simulink model "EndEffectorVSCube_v2"  (Simulink 7.4)
settings: Solver=FixedStepDiscrete  StartTime=0.0  StopTime=80  FixedStep=dt  RelTol=1e-3
InitFcn:
  | start_EEVSCube2
undefined symbols (not defined in the file or in its folder): DiscIntNeverNeededParam, dt, mesh_A, mesh_B
libraries: simulink x2, dspsigops x1
settings Model: Creator=SIMONE  LastModifiedBy=Administrator
settings SolverCC: PositivePriorityOrder=on
settings DataIOCC: LimitDataPoints=off  SaveOutput=off  SignalLogging=off
settings RTWCC: GenerateMakefile=off

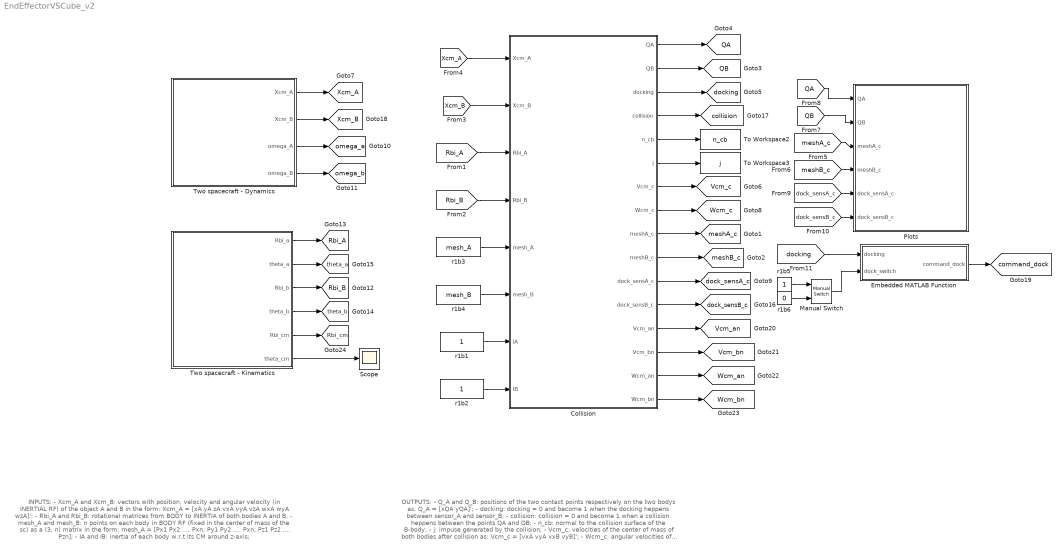
== system EndEffectorVSCube_v2 ==
  note: INPUTS:
      | - Xcm_A and Xcm_B: vectors with position, velocity and angular velocity (in INERTIAL RF)
      |                                        of the object A and B in the form:
      |                                        Xcm_A = [xA yA zA vxA vyA vzA wxA wyA wzA]';
      | - Rbi_A and Rbi_B: rotational matrices from BODY to INERTIA of both bodies A and B;
      | - mesh_A and mesh_B: n points on each body in BODY RF (fixed in the center of mass
      |                                          of the sc) as a (3, n) matrix in the form:
      |                                          mesh_A = [Px1 Px2 .... Pxn;
      |                                                             Py1 Py2 .... Pxn;
      |                                                             Pz1 Pz2 .... Pzn];
      | - IA and IB: inertia of each body w.r.t its CM around z-axis;
  note: OUTPUTS:
      | - Q_A and Q_B: positions of the two contact points respectively on the two bodys as,
      |                              Q_A = [xQA yQA]';
      | - docking: docking = 0 and become 1 when the docking heppens between sensor_A and sensor_B;
      | - collision: collision = 0 and become 1 when a collision heppens between the points QA and QB;
      | - n_cb: normal to the collision surface of the B-body;
      | - j: impuse generated by the collision;
      | - Vcm_c: velocities of the center of mass of both bodies after collision as:
      |                  Vcm_c = [vxA vyA vxB vyB]';
      | - Wcm_c: angular velocities of the center of mass of both bodies after collision as:
      |                    Wcm_c = [wxA wyA wxB wyB]'.
      | - meshA_c and meshB_c: n points on each body in INERTIAL RF propagated during the simulation,
      |                                                     as a (1, 3*n) vector in the form:
      |                                                      pointsA_c = [Px1 Py1 Px2 Py2 .... Pxn Pyn];
      | - dock_sensA_c and dock_sensB_c: position of the docking sensors on A and B in INERTIAL RF while simulation is running;
  Collision : Subsystem  mask{mA=1e6, mB=1, sigma=0.01, sigma_dock=0.1, dotsigma_dock=1, dock_sensA=[0.5 0 0]', dock_sensB=[-0.5 0 0]', epsilon=1}
      mask prompts: mA "Mass of body A [Kg]"; mB "Mass of body B [Kg]"; sigma "Minimum distance for contact [m]"; sigma_dock "Minimum distance for docking (must be greater than contact distance) [m]"; dotsigma_dock "Maximum relative velocity for docking [m/s]"; dock_sensA "Docking sensor position (Body RF) on body A (as [x y z]') [m]"; dock_sensB "Docking sensor position (Body RF) on body B (as [x y z]') [m]"; epsilon "Coefficent of restitution"
      mask help: This block implements collision detection and responce for two rigid bodies of general shapes.
      mask init:
      | ma_mb = [mA; 
      |          mB];
      mask Display:
      | image(imread('collision.jpeg'))
      | color('red');
      | disp('Collision \n Detection and Responce \n v.1.0.9')
      | port_label('input',1,'Xcm_A')
      | port_label('input',2,'Xcm_B')
      | port_label('input',3,'Rbi_A')
      | port_label('input',4,'Rbi_B')
      | port_label('input',5,'mesh_A')
      | port_label('input',6,'mesh_B')
      | port_label('input',7,'IA')
      | port_label('input',8,'IB')
      | 
      | port_label('output',1,'QA')
      | port_label('output',2,'QB')
      | port_label('output',3,'docking')
      | port_label('output',4,'collision')
      | port_label('output',5,'n_cb')
      | port_label('output',6,'j')
      | port_label('output',7,'Vcm_c')
      | port_label('output',8,'Wcm_c')
      | port_label('output',9,'meshA_c')
      | port_label('output',10,'meshB_c')
      | port_label('output',11,'dock_sensA_c')
      | port_label('output',12,'dock_sensB_c')
      | port_label('output',13,'Vcm_an')
      | port_label('output',14,'Vcm_bn')
      | port_label('output',15,'Wcm_an')
      | port_label('output',16,'Wcm_bn')
  Embedded MATLAB Function : Stateflow chart  TreatAsAtomicUnit=on
  Manual Switch : simulink/Signal Routing/Manual Switch  SystemSampleTime=-1  sw=1  action=0  varsize=off
  Plots : Subsystem
  Scope : Scope
      settings: TimeRange=3  YMin=-1  YMax=1.5  SaveName=ScopeData3
  To Workspace2 : ToWorkspace  VariableName=n_cb  SampleTime=-1  SaveFormat=Array
  To Workspace3 : ToWorkspace  VariableName=j  SampleTime=-1  SaveFormat=Array
  Two spacecraft - Dynamics : Subsystem
  Two spacecraft - Kinematics : Subsystem
  r1b1 : Constant
  r1b2 : Constant
  r1b3 : Constant  Value=mesh_A
  r1b4 : Constant  Value=mesh_B
  r1b5 : Constant
  r1b6 : Constant  Value=0
  tag scope: QA=global, QB=global, Rbi_A=global, Rbi_B=global, Rbi_cm=global, Vcm_an=global, Vcm_bn=global, Vcm_c=global, Wcm_an=global, Wcm_bn=global, Wcm_c=global, Xcm_A=global, Xcm_B=global, collision=global, command_dock=global, dock_sensA_c=global, dock_sensB_c=global, docking=global, meshA_c=global, meshB_c=global, omega_a=global, omega_b=global, theta_a=global, theta_b=global
  wires:
  Collision/1(QA) -> [QA]
  Collision/2(QB) -> [QB]
  Collision/3(docking) -> [docking]
  Two spacecraft - Dynamics/3(omega_A) -> [omega_a]
  Two spacecraft - Dynamics/4(omega_B) -> [omega_b]
  Two spacecraft - Dynamics/1(Xcm_A) -> [Xcm_A]
  Two spacecraft - Kinematics/3(Rbi_b) -> [Rbi_B]
  Two spacecraft - Kinematics/1(Rbi_a) -> [Rbi_A]
  Two spacecraft - Kinematics/2(theta_a) -> [theta_a]
  Two spacecraft - Kinematics/4(theta_b) -> [theta_b]
  Collision/6(j) -> To Workspace3/1
  Collision/4(collision) -> [collision]
  Two spacecraft - Dynamics/2(Xcm_B) -> [Xcm_B]
  [Xcm_A] -> Collision/1(Xcm_A)
  [Xcm_B] -> Collision/2(Xcm_B)
  [Rbi_A] -> Collision/3(Rbi_A)
  [Rbi_B] -> Collision/4(Rbi_B)
  r1b3/1 -> Collision/5(mesh_A)
  r1b4/1 -> Collision/6(mesh_B)
  Collision/5(n_cb) -> To Workspace2/1
  Collision/7(Vcm_c) -> [Vcm_c]
  Collision/8(Wcm_c) -> [Wcm_c]
  Collision/9(meshA_c) -> [meshA_c]
  Collision/10(meshB_c) -> [meshB_c]
  [QA] -> Plots/1(QA)
  [QB] -> Plots/2(QB)
  [meshA_c] -> Plots/3(meshA_c)
  [meshB_c] -> Plots/4(meshB_c)
  Collision/11(dock_sensA_c) -> [dock_sensA_c]
  Collision/12(dock_sensB_c) -> [dock_sensB_c]
  [dock_sensA_c] -> Plots/5(dock_sensA_c)
  [dock_sensB_c] -> Plots/6(dock_sensB_c)
  r1b1/1 -> Collision/7(IA)
  r1b2/1 -> Collision/8(IB)
  [docking] -> Embedded MATLAB Function/1(docking)
  Embedded MATLAB Function/1(command_dock) -> [command_dock]
  Manual Switch/1 -> Embedded MATLAB Function/2(dock_switch)
  r1b5/1 -> Manual Switch/1
  r1b6/1 -> Manual Switch/2
  Collision/13(Vcm_an) -> [Vcm_an]
  Collision/14(Vcm_bn) -> [Vcm_bn]
  Collision/15(Wcm_an) -> [Wcm_an]
  Collision/16(Wcm_bn) -> [Wcm_bn]
  Two spacecraft - Kinematics/5(Rbi_cm) -> [Rbi_cm]
  Two spacecraft - Kinematics/6(theta_cm) -> Scope/1

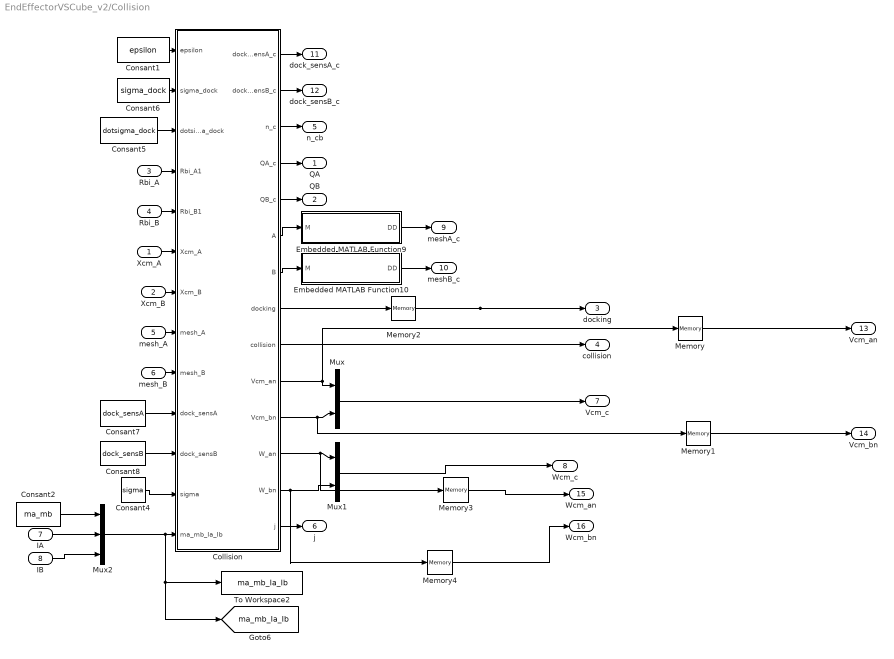
== system EndEffectorVSCube_v2/Collision ==
  Xcm_A : Inport
  Xcm_B : Inport  Port=2
  Rbi_A : Inport  Port=3
  Rbi_B : Inport  Port=4
  mesh_A : Inport  Port=5
  mesh_B : Inport  Port=6
  IA : Inport  Port=7
  IB : Inport  Port=8
  Collision : Stateflow chart  TreatAsAtomicUnit=on
  Consant1 : Constant  Value=epsilon
  Consant2 : Constant  Value=ma_mb
  Consant4 : Constant  Value=sigma
  Consant5 : Constant  Value=dotsigma_dock
  Consant6 : Constant  Value=sigma_dock
  Consant7 : Constant  Value=dock_sensA
  Consant8 : Constant  Value=dock_sensB
  Embedded MATLAB Function10 : Stateflow chart  TreatAsAtomicUnit=on
  Embedded MATLAB Function9 : Stateflow chart  TreatAsAtomicUnit=on
  Memory{,1,3..4} (4 alike) : Memory  X0=zeros(3,1)
  Memory2 : Memory
  Mux : Mux  Inputs=2
  Mux1 : Mux  Inputs=2
  Mux2 : Mux  Inputs=3
  To Workspace2 : ToWorkspace  VariableName=ma_mb_Ia_Ib  SampleTime=-1  SaveFormat=Array
  QA : Outport
  QB : Outport  Port=2
  docking : Outport  Port=3
  collision : Outport  Port=4
  n_cb : Outport  Port=5
  j : Outport  Port=6
  Vcm_c : Outport  Port=7
  Wcm_c : Outport  Port=8
  meshA_c : Outport  Port=9
  meshB_c : Outport  Port=10
  dock_sensA_c : Outport  Port=11
  dock_sensB_c : Outport  Port=12
  Vcm_an : Outport  Port=13
  Vcm_bn : Outport  Port=14
  Wcm_an : Outport  Port=15
  Wcm_bn : Outport  Port=16
  tag scope: ma_mb_Ia_Ib=global
  wires:
  Embedded MATLAB Function9/1(DD) -> meshA_c/1
  Embedded MATLAB Function10/1(DD) -> meshB_c/1
  Collision/6(A) -> Embedded MATLAB Function9/1(M)
  Collision/7(B) -> Embedded MATLAB Function10/1(M)
  Rbi_B/1 -> Collision/5(Rbi_B1)
  Xcm_A/1 -> Collision/6(Xcm_A)
  mesh_A/1 -> Collision/8(mesh_A)
  mesh_B/1 -> Collision/9(mesh_B)
  Collision/3(n_c) -> n_cb/1
  Collision/8(docking) -> Memory2/1
  Collision/10(Vcm_an) -> Mux/1, Memory/1
  Collision/13(W_bn) -> Mux1/2, Memory4/1
  Collision/14(j) -> j/1
  Collision/9(collision) -> collision/1
  Mux/1 -> Vcm_c/1
  Mux1/1 -> Wcm_c/1
  Collision/4(QA_c) -> QA/1
  Collision/5(QB_c) -> QB/1
  Collision/11(Vcm_bn) -> Memory1/1, Mux/2
  Collision/12(W_an) -> Memory3/1, Mux1/1
  Xcm_B/1 -> Collision/7(Xcm_B)
  Collision/2(dock_sensB_c) -> dock_sensB_c/1
  Collision/1(dock_sensA_c) -> dock_sensA_c/1
  Consant4/1 -> Collision/12(sigma)
  Consant5/1 -> Collision/3(dotsigma_dock)
  Rbi_A/1 -> Collision/4(Rbi_A1)
  Consant6/1 -> Collision/2(sigma_dock)
  Consant7/1 -> Collision/10(dock_sensA)
  Consant8/1 -> Collision/11(dock_sensB)
  Consant1/1 -> Collision/1(epsilon)
  Mux2/1 -> Collision/13(ma_mb_Ia_Ib), To Workspace2/1, [ma_mb_Ia_Ib]
  Consant2/1 -> Mux2/1
  IA/1 -> Mux2/2
  IB/1 -> Mux2/3
  Memory/1 -> Vcm_an/1
  Memory1/1 -> Vcm_bn/1
  Memory3/1 -> Wcm_an/1
  Memory4/1 -> Wcm_bn/1
  Memory2/1 -> docking/1

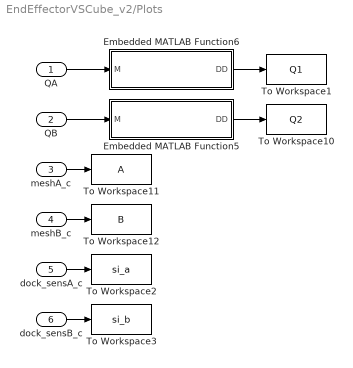
== system EndEffectorVSCube_v2/Plots ==
  QA : Inport
  QB : Inport  Port=2
  meshA_c : Inport  Port=3
  meshB_c : Inport  Port=4
  dock_sensA_c : Inport  Port=5
  dock_sensB_c : Inport  Port=6
  Embedded MATLAB Function5 : Stateflow chart  TreatAsAtomicUnit=on
  Embedded MATLAB Function6 : Stateflow chart  TreatAsAtomicUnit=on
  To Workspace1 : ToWorkspace  VariableName=Q1  SampleTime=-1  SaveFormat=Array
  To Workspace10 : ToWorkspace  VariableName=Q2  SampleTime=-1  SaveFormat=Array
  To Workspace11 : ToWorkspace  VariableName=A  SampleTime=-1  SaveFormat=Array
  To Workspace12 : ToWorkspace  VariableName=B  SampleTime=-1  SaveFormat=Array
  To Workspace2 : ToWorkspace  VariableName=si_a  SampleTime=-1  SaveFormat=Array
  To Workspace3 : ToWorkspace  VariableName=si_b  SampleTime=-1  SaveFormat=Array
  wires:
  Embedded MATLAB Function6/1(DD) -> To Workspace1/1
  Embedded MATLAB Function5/1(DD) -> To Workspace10/1
  QA/1 -> Embedded MATLAB Function6/1(M)
  QB/1 -> Embedded MATLAB Function5/1(M)
  meshB_c/1 -> To Workspace12/1
  meshA_c/1 -> To Workspace11/1
  dock_sensA_c/1 -> To Workspace2/1
  dock_sensB_c/1 -> To Workspace3/1

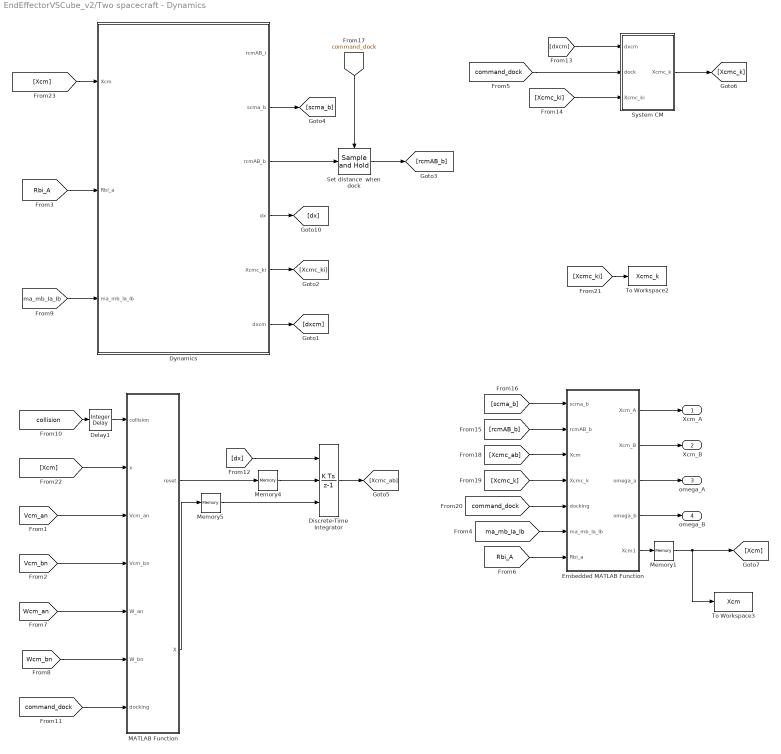
== system EndEffectorVSCube_v2/Two spacecraft - Dynamics ==
  Delay1 : simulink/Discrete/Integer Delay  vinit=0  samptime=-1  NumDelays=1
  Discrete-Time Integrator : DiscreteIntegrator  ExternalReset=rising  InitialConditionSource=external  SampleTime=dt  ICPrevOutput=DiscIntNeverNeededParam  ICPrevScaledInput=DiscIntNeverNeededParam
  Dynamics : Stateflow chart  TreatAsAtomicUnit=on
  Embedded MATLAB Function : Stateflow chart  TreatAsAtomicUnit=on
  MATLAB Function : Stateflow chart  TreatAsAtomicUnit=on
  Memory1 : Memory  X0=zeros(10,1)
  Memory4 : Memory
  Memory5 : Memory  X0=[-1, 0, 0, 0, 0, 2.5*2, 0, -0.2, 0, -0.2]'
  Set distance  when dock : dspsigops/Sample and Hold  SystemSampleTime=-1  trig=Rising edge  initCond=0  latchinput=off
  System CM : Subsystem
  To Workspace2 : ToWorkspace  VariableName=Xcmc_k  SampleTime=-1  SaveFormat=Array
  To Workspace3 : ToWorkspace  VariableName=Xcm  SampleTime=-1  SaveFormat=Array
  Xcm_A : Outport  PortDimensions=[9,1]
  Xcm_B : Outport  Port=2  PortDimensions=[9,1]
  omega_A : Outport  Port=3
  omega_B : Outport  Port=4
  wires:
  [Rbi_A] -> Dynamics/2(Rbi_a)
  Embedded MATLAB Function/1(Xcm_A) -> Xcm_A/1
  Embedded MATLAB Function/2(Xcm_B) -> Xcm_B/1
  MATLAB Function/2(X) -> Memory5/1
  Memory5/1 -> Discrete-Time Integrator/3
  MATLAB Function/1(reset) -> Memory4/1
  Embedded MATLAB Function/3(omega_a) -> omega_A/1
  Embedded MATLAB Function/4(omega_b) -> omega_B/1
  [Vcm_an] -> MATLAB Function/3(Vcm_an)
  [Vcm_bn] -> MATLAB Function/4(Vcm_bn)
  [collision] -> Delay1/1
  Memory4/1 -> Discrete-Time Integrator/2
  [Wcm_an] -> MATLAB Function/5(W_an)
  [Wcm_bn] -> MATLAB Function/6(W_bn)
  [ma_mb_Ia_Ib] -> Dynamics/3(ma_mb_Ia_Ib)
  [ma_mb_Ia_Ib] -> Embedded MATLAB Function/6(ma_mb_Ia_Ib)
  Delay1/1 -> MATLAB Function/1(collision)
  [command_dock] -> System CM/2(dock)
  [Rbi_A] -> Embedded MATLAB Function/7(Rbi_a)
  Embedded MATLAB Function/5(Xcm1) -> Memory1/1
  Dynamics/4(dx) -> [dx]
  [dx] -> Discrete-Time Integrator/1
  Dynamics/6(dxcm) -> [dxcm]
  [dxcm] -> System CM/1(dxcm)
  Dynamics/5(Xcmc_ki) -> [Xcmc_ki]
  [Xcmc_ki] -> System CM/3(Xcmc_ki)
  [rcmAB_b] -> Embedded MATLAB Function/2(rcmAB_b)
  [scma_b] -> Embedded MATLAB Function/1(scma_b)
  Dynamics/2(scma_b) -> [scma_b]
  [command_dock] -> Set distance  when dock/Trigger
  Set distance  when dock/1 -> [rcmAB_b]
  Dynamics/3(rcmAB_b) -> Set distance  when dock/1
  Discrete-Time Integrator/1 -> [Xcmc_ab]
  [Xcmc_ab] -> Embedded MATLAB Function/3(Xcm)
  System CM/1(Xcmc_k) -> [Xcmc_k]
  [Xcmc_k] -> Embedded MATLAB Function/4(Xcmc_k)
  [command_dock] -> Embedded MATLAB Function/5(docking)
  [Xcmc_ki] -> To Workspace2/1
  [Xcm] -> MATLAB Function/2(x)
  [Xcm] -> Dynamics/1(Xcm)
  Memory1/1 -> [Xcm], To Workspace3/1
  [command_dock] -> MATLAB Function/7(docking)

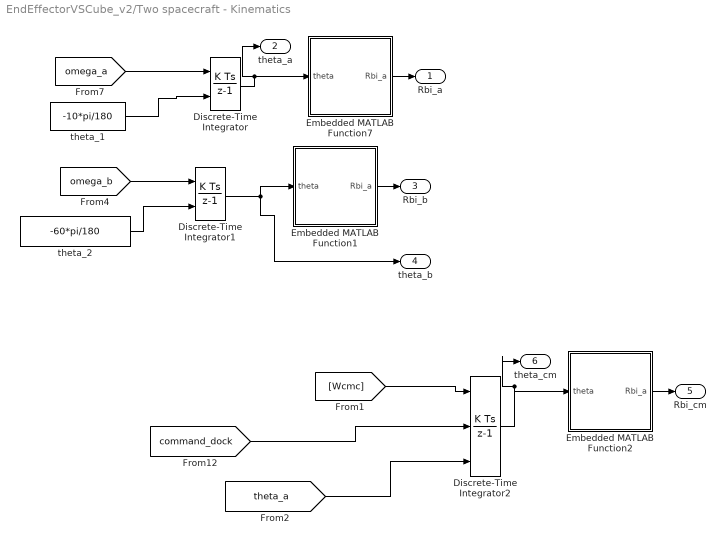
== system EndEffectorVSCube_v2/Two spacecraft - Kinematics ==
  Discrete-Time Integrator : DiscreteIntegrator  InitialConditionSource=external  SampleTime=dt  ICPrevOutput=DiscIntNeverNeededParam  ICPrevScaledInput=DiscIntNeverNeededParam
  Discrete-Time Integrator1 : DiscreteIntegrator  InitialConditionSource=external  SampleTime=dt  ICPrevOutput=DiscIntNeverNeededParam  ICPrevScaledInput=DiscIntNeverNeededParam
  Discrete-Time Integrator2 : DiscreteIntegrator  ExternalReset=rising  InitialConditionSource=external  SampleTime=dt  ICPrevOutput=DiscIntNeverNeededParam  ICPrevScaledInput=DiscIntNeverNeededParam
  Embedded MATLAB Function1 : Stateflow chart  TreatAsAtomicUnit=on
  Embedded MATLAB Function2 : Stateflow chart  TreatAsAtomicUnit=on
  Embedded MATLAB Function7 : Stateflow chart  TreatAsAtomicUnit=on
  theta_1 : Constant  Value=-10*pi/180
  theta_2 : Constant  Value=-60*pi/180
  Rbi_a : Outport  PortDimensions=[2,2]
  theta_a : Outport  Port=2
  Rbi_b : Outport  Port=3  PortDimensions=[2,2]
  theta_b : Outport  Port=4
  Rbi_cm : Outport  Port=5  PortDimensions=[2,2]
  theta_cm : Outport  Port=6
  wires:
  [omega_a] -> Discrete-Time Integrator/1
  theta_1/1 -> Discrete-Time Integrator/2
  Embedded MATLAB Function7/1(Rbi_a) -> Rbi_a/1
  Embedded MATLAB Function1/1(Rbi_a) -> Rbi_b/1
  Discrete-Time Integrator/1 -> theta_a/1, Embedded MATLAB Function7/1(theta)
  Discrete-Time Integrator1/1 -> Embedded MATLAB Function1/1(theta), theta_b/1
  [omega_b] -> Discrete-Time Integrator1/1
  theta_2/1 -> Discrete-Time Integrator1/2
  [Wcmc] -> Discrete-Time Integrator2/1
  Embedded MATLAB Function2/1(Rbi_a) -> Rbi_cm/1
  Discrete-Time Integrator2/1 -> Embedded MATLAB Function2/1(theta), theta_cm/1
  [command_dock] -> Discrete-Time Integrator2/2
  [theta_a] -> Discrete-Time Integrator2/3

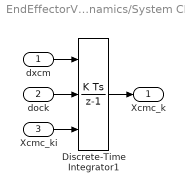
== system EndEffectorVSCube_v2/Two spacecraft - Dynamics/System CM ==
  dxcm : Inport
  dock : Inport  Port=2
  Xcmc_ki : Inport  Port=3
  Discrete-Time Integrator1 : DiscreteIntegrator  ExternalReset=rising  InitialConditionSource=external  SampleTime=dt  ICPrevOutput=DiscIntNeverNeededParam  ICPrevScaledInput=DiscIntNeverNeededParam
  Xcmc_k : Outport
  wires:
  dxcm/1 -> Discrete-Time Integrator1/1
  dock/1 -> Discrete-Time Integrator1/2
  Discrete-Time Integrator1/1 -> Xcmc_k/1
  Xcmc_ki/1 -> Discrete-Time Integrator1/3

== matlab function Two spacecraft - Dynamics/Embedded MATLAB Function ==
  data: scma_b input double; Xcm_A output double; Xcm_B output double; omega_a output double; omega_b output double; Xcm1 output double; rcmAB_b input double; Xcm input double; Xcmc_k input double; docking input double; ma_mb_Ia_Ib input double; Rbi_a input double
function [Xcm_A, Xcm_B,omega_a,omega_b,Xcm1]  = fcn(scma_b,rcmAB_b,Xcm,Xcmc_k, docking, ma_mb_Ia_Ib,Rbi_a)
ma=ma_mb_Ia_Ib(1);
mb=ma_mb_Ia_Ib(2);
Ia=ma_mb_Ia_Ib(3);
Ib=ma_mb_Ia_Ib(4);
% Xcm_B=zeros(9,1);
% Xcm_A=zeros(9,1);

% omega_a=0;
% omega_b=0;
%rcmAB_b=zeros(3,1);

omega_a=Xcm(5);
omega_b=Xcm(10);

xyA = Xcm(1:2);
dxyA = Xcm(3:4);
wA = Xcm(5);

xyB= Xcm(6:7);
dxyB = Xcm(8:9);
wB = Xcm(10);


Xcm_A = [xyA;
         0;
         dxyA;
         0;
         0;
         0;
         wA];
     
Xcm_B = [xyB;
          0;
          dxyB;
          0;
          0;
          0;
          wB];
      
      Xcm1=Xcm;
      
if(docking == 1)
    
    rcm_tot=Xcmc_k(1:2,1);
    vcm_tot=[Xcmc_k(3:4,1); 0];
    %scma_b=[0.5 0 0]';
    wcm_tot=[0 0 Xcmc_k(5)]';
   
    Rbi_a_3=[Rbi_a zeros(2,1)
           0 0 1];
    scma_i=Rbi_a_3*scma_b;
    %body A   
    
    xya=rcm_tot+Rbi_a*scma_b(1:2,1);
    dxya=vcm_tot+cross(wcm_tot,scma_i);
    wa=wcm_tot(3);
    
    %body B
    rcmAB_i=Rbi_a_3*rcmAB_b;
    xyb=xya+rcmAB_i(1:2,1);
    dxyb=dxya+cross(wcm_tot,rcmAB_i);
    wb=wa;
    
    
    
    Xcm_A = [xya;
         0;
         dxya;
         0;
         0;
         wa];
    
       Xcm_B = [xyb;
         0;
         dxyb;
         0;
         0;
         wb];
     
     Xcm1=[xya;
         dxya(1:2);
         wa;
         xyb;
         dxyb(1:2);
         wb];
 omega_a=wa;
omega_b=wb;
    

   
end

== matlab function Collision/Collision ==
  data: epsilon input double; dock_sensA_c output double; dock_sensB_c output double; n_c output double; QA_c output double; QB_c output double; sigma_dock input double; dotsigma_dock input double; Rbi_A1 input double; Rbi_B1 input double; A output double; B output double; Xcm_A input double; Xcm_B input double; mesh_A input double; mesh_B input double; dock_sensA input double; dock_sensB input double; sigma input double; docking output double; ma_mb_Ia_Ib input double; collision output double; Vcm_an output double; Vcm_bn output double; W_an output double; W_bn output double; j output double
function [dock_sensA_c,dock_sensB_c,n_c,QA_c,QB_c,A,B,docking,collision,Vcm_an,Vcm_bn,W_an,W_bn,j] = fcn(epsilon,sigma_dock,dotsigma_dock,Rbi_A1,Rbi_B1,Xcm_A,Xcm_B,mesh_A,mesh_B,dock_sensA,dock_sensB,sigma,ma_mb_Ia_Ib)

[dock_sensA_c,dock_sensB_c,n_c,QA_c,QB_c,A,B,docking,collision,Vcm_an,Vcm_bn,W_an,W_bn,j] = collision_function(epsilon,sigma_dock,dotsigma_dock,Rbi_A1,Rbi_B1,Xcm_A,Xcm_B,mesh_A,mesh_B,dock_sensA,dock_sensB,sigma,ma_mb_Ia_Ib);

== matlab function Two spacecraft - Kinematics/Embedded MATLAB Function1 ==
  data: theta input double; Rbi_a output double
function Rbi_a   = fcn(theta)
%%Defining point 
Rib=[cos(theta) sin(theta)
    -sin(theta) cos(theta)];
Rbi_a=Rib';

== matlab function Two spacecraft - Dynamics/Dynamics ==
  data: rcmAB_i output double; scma_b output double; rcmAB_b output double; Xcm input double; Rbi_a input double; dx output double; Xcmc_ki output double; ma_mb_Ia_Ib input double; dxcm output double
function [rcmAB_i,scma_b,rcmAB_b, dx,Xcmc_ki,dxcm]  = fcn(Xcm, Rbi_a, ma_mb_Ia_Ib)

ma=ma_mb_Ia_Ib(1);
mb=ma_mb_Ia_Ib(2);
Ia=ma_mb_Ia_Ib(3);
Ib=ma_mb_Ia_Ib(4);
rcmAB_b=zeros(3,1);

scma_b=zeros(3,1);


dt=0.01;

%size of the dynamics
dx=zeros(10,1);
dxcm=zeros(5,1);

g = -0.81*0;

%define variable for A

x_a=Xcm(1);
y_a=Xcm(2);
vx_a = Xcm(3);
vy_a = Xcm(4);
w_a=Xcm(5);

% define variable for B
x_b=Xcm(6);
y_b=Xcm(7);
vx_b = Xcm(8);
vy_b = Xcm(9);
w_b=Xcm(10);
 
dx(1) = vx_a;
dx(2) = vy_a;
dx(3) = 0;
dx(4) = 0+g;
dx(5) = 0;
dx(6) = vx_b;
dx(7) = vy_b;
dx(8) = 0;
dx(9) = 0+g;
dx(10) =0;



 
%%define the total center of mass and velocity

Xcm_a=[x_a y_a 0]';
Vcm_a=[vx_a vy_a 0]';
W_a=[0 0 w_a]';

Xcm_b=[x_b y_b 0]';
Vcm_b=[vx_b vy_b 0]';
W_b=[0 0 w_b]';


Rbi_a_3 = [Rbi_a zeros(2,1)
           0 0 1];
rcmAB_i=(Xcm_b - Xcm_a);

rcmAB_b = Rbi_a_3'*rcmAB_i;

% center of mass generation

Xcmc_k=(ma*Xcm_a+mb*Xcm_b)/(ma+mb);
Vcmc_k=(ma*Vcm_a+mb*Vcm_b)/(ma+mb);

Itot=Ia+Ib;
Wcmc_k=inv(Itot)*(Ia*W_a+Ib*W_b+cross(Xcm_a,ma*Vcm_a)+cross(Xcm_b,ma*Vcm_b)-cross(Xcmc_k,(ma+mb)*Vcmc_k));

%Wcmc_k=(Ia*W_a(3)+Ib*W_b(3))/(Ia+Ib);

 Xcmc_ki=[Xcmc_k(1:2)
         Vcmc_k(1:2)
       Wcmc_k(3)];




scma_b=Rbi_a_3'*(Xcm_a-Xcmc_k);
%scma_b=(Xcm_a-Xcmc_k);


dxcm(1) = Vcmc_k(1);
dxcm(2) = Vcmc_k(2);
dxcm(3) = 0;
dxcm(4) = 0;
dxcm(5) = 0;

== matlab function Plots/Embedded MATLAB Function5 ==
  data: M input double; DD output double
function DD=fcn(M)

[m,n] = size(M);
a = zeros(n*m,1);
MM=zeros(n*m,1);
i=1;
for mm=0:m:n*m-1
for j=1:1:m
    a(j+mm,1)=M(j,i); 
end
i=i+1;
end
DD=a;

== matlab function Plots/Embedded MATLAB Function6 ==
  data: M input double; DD output double
function DD=fcn(M)

[m,n] = size(M);
a = zeros(n*m,1);
MM=zeros(n*m,1);
i=1;
for mm=0:m:n*m-1
for j=1:1:m
    a(j+mm,1)=M(j,i); 
end
i=i+1;
end
DD=a;

== matlab function Two spacecraft - Kinematics/Embedded MATLAB Function7 ==
  data: theta input double; Rbi_a output double
function Rbi_a   = fcn(theta)
%%Defining point 
Rib=[cos(theta) sin(theta)
    -sin(theta) cos(theta)];
Rbi_a=Rib';

== matlab function Collision/Embedded MATLAB Function9 ==
  data: M input double; DD output double
function DD=fcn(M)

[m,n] = size(M);
a = zeros(n*m,1);
MM=zeros(n*m,1);
i=1;
for mm=0:m:n*m-1
for j=1:1:m
    a(j+mm,1)=M(j,i); 
end
i=i+1;
end
DD=a;

== matlab function Collision/Embedded MATLAB Function10 ==
  data: M input double; DD output double
function DD=fcn(M)

[m,n] = size(M);
a = zeros(n*m,1);
MM=zeros(n*m,1);
i=1;
for mm=0:m:n*m-1
for j=1:1:m
    a(j+mm,1)=M(j,i); 
end
i=i+1;
end
DD=a;

== matlab function Embedded MATLAB Function ==
  data: docking input double; command_dock output double; dock_switch input double
function command_dock  = fcn(docking, dock_switch)
persistent k
if isempty(k)
    k=0;
end
command_dock=0;


if docking == 1 && dock_switch == 1
    command_dock = 1;
    k=5;
else
    command_dock = 0;
end

% 
%  if docking == 1 && dock_switch == 1
% %     command_dock = 1;
%      k=5;
% %     command_dock = 0;
%  end
% 
%  if (k>2)
%      command_dock = 1;
%  end

== matlab function Two spacecraft - Dynamics/MATLAB Function ==
  data: reset output double; collision input double; X output double; x input double; Vcm_an input double; Vcm_bn input double; W_an input double; W_bn input double; docking input double
function [reset,X] = fcn(collision,x,Vcm_an,Vcm_bn,W_an,W_bn,docking)
%#eml

X=zeros(10,1);
if(docking==1)
    X=x;
    reset=0;
else
    if(collision==1)
        x(3)=Vcm_an(1);
        x(4)=Vcm_an(2);
        x(5)=W_an(3);
        
        x(8)=Vcm_bn(1);
        x(9)=Vcm_bn(2);
        x(10)=W_bn(3);
        W_an(3)
        W_bn(3)
        reset=1;
    else
        reset=0;
        
    end
    
    
    
    
    X=x;
end

== matlab function Two spacecraft - Kinematics/Embedded MATLAB Function2 ==
  data: theta input double; Rbi_a output double
function Rbi_a   = fcn(theta)
%%Defining point 
Rib=[cos(theta) sin(theta)
    -sin(theta) cos(theta)];
Rbi_a=Rib';
